simulink library "propertySpecificationOperatorLib"  (Simulink 7.6)
settings: Solver=FixedStepDiscrete  StartTime=0.0  StopTime=10.0  FixedStep=Auto  RelTol=1e-3
libraries: simulink x3, sldvlib x2
settings Model: Creator=itoy  LastModifiedBy=itoy

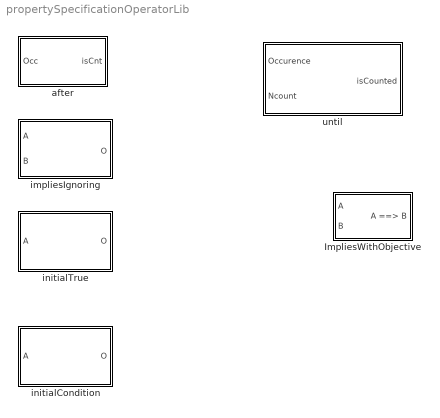
== system propertySpecificationOperatorLib ==
  ImpliesWithObjective : Subsystem
      mask Type: Design Verifier Implies
      mask Description:
      | Tests whether the first input implies the second.  Outputs false
      | when first input is true and second input is false, otherwise
      | outputs true.
      mask Help: helpview(fullfile(docroot,'toolbox','sldv','sldv.map'),'implies')
      mask Display: disp(' ')
  after : Subsystem  mask(After block){TickCount=1}
      mask help:
      | This is an after block.
      | If Occurence are true for successive Ncount time steps, output will be true.
      mask Help: This is a counter block.
      mask Display: fprintf('\nAfter')
  impliesIgnoring : Subsystem  mask{DelayCount=4}
      mask prompts: DelayCount "Delay Count"
      mask Display: fprintf('Implies ignoring\n initial %d steps',DelayCount)
  initialCondition : Subsystem  mask(ignoreInitSteps){DelayCount=4}
      mask prompts: DelayCount "Delay Count"
      mask Display: fprintf('True after \n initial %d steps',DelayCount)
  initialTrue : Subsystem  mask(ignoreInitSteps){DelayCount=5}
      mask prompts: DelayCount "Delay Count"
      mask Display: fprintf('True for \n initial %d steps',DelayCount)
  until : Subsystem  TreatAsAtomicUnit=on
      mask Type: After block
      mask Description:
      | This is an after block.
      | If Occurence are true for successive Ncount time steps, output will be true.
      mask Help: This is a counter block.
      mask Display: fprintf('Until')

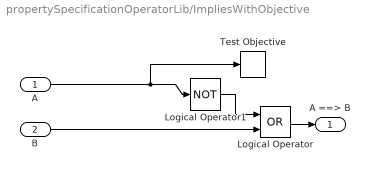
== system propertySpecificationOperatorLib/ImpliesWithObjective ==
  A : Inport
  B : Inport  Port=2
  Logical Operator : Logic  Operator=OR  AllPortsSameDT=off  OutDataTypeStr=boolean
  Logical Operator1 : Logic  Operator=NOT  AllPortsSameDT=off  OutDataTypeStr=boolean
  Test Objective : sldvlib/Test Objective  SystemSampleTime=-1  enabled=on  customAVTBlockType=Test Objective  intervals=true  dispValues=on  outEnabled=off
      settings: AttributesFormatString=%<intervals>
  A ==> B : Outport
  wires:
  Logical Operator1/1 -> Logical Operator/1
  A/1 -> Logical Operator1/1, Test Objective/1
  Logical Operator/1 -> A ==> B/1
  B/1 -> Logical Operator/2

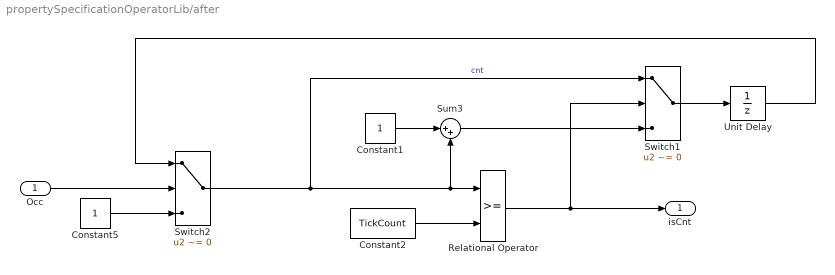
== system propertySpecificationOperatorLib/after ==
  Occ : Inport  OutDataTypeStr=boolean
  Constant1 : Constant  OutDataTypeStr=Inherit: Inherit via back propagation
  Constant2 : Constant  Value=TickCount  OutDataTypeStr=Inherit: Inherit via back propagation
  Constant5 : Constant  OutDataTypeStr=Inherit: Inherit via back propagation
  Relational Operator : RelationalOperator  OutDataTypeStr=boolean
  Sum3 : Sum  Inputs=|++  OutDataTypeStr=Inherit: Inherit via back propagation
  Switch1 : Switch  Criteria=u2 ~= 0  OutDataTypeStr=Inherit: Inherit via back propagation
  Switch2 : Switch  Criteria=u2 ~= 0  OutDataTypeStr=uint8
  Unit Delay : UnitDelay  X0=1  SampleTime=-1
      settings: AttributesFormatString=Init = %<X0>
  isCnt : Outport
  wires:
  Relational Operator/1 -> isCnt/1, Switch1/2
  Constant2/1 -> Relational Operator/2
  Switch2/1 -> Sum3/2, Relational Operator/1, Switch1/1  "cnt"
  Occ/1 -> Switch2/2
  Constant5/1 -> Switch2/3
  Constant1/1 -> Sum3/1
  Unit Delay/1 -> Switch2/1
  Switch1/1 -> Unit Delay/1
  Sum3/1 -> Switch1/3

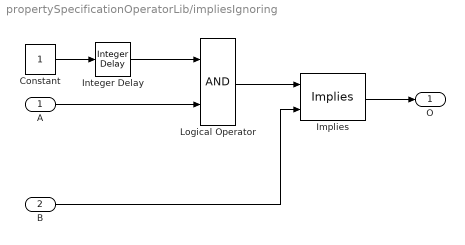
== system propertySpecificationOperatorLib/impliesIgnoring ==
  A : Inport
  B : Inport  Port=2
  Constant : Constant  OutDataTypeStr=boolean
  Implies : sldvlib/Implies  SystemSampleTime=-1
  Integer Delay : simulink/Discrete/Integer Delay  NumDelays=DelayCount  InputProcessing=Inherited  vinit=0  samptime=-1
  Logical Operator : Logic  AllPortsSameDT=off  OutDataTypeStr=boolean
  O : Outport
  wires:
  Implies/1 -> O/1
  Logical Operator/1 -> Implies/1
  Constant/1 -> Integer Delay/1
  Integer Delay/1 -> Logical Operator/1
  A/1 -> Logical Operator/2
  B/1 -> Implies/2

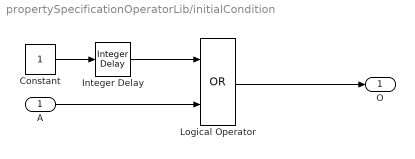
== system propertySpecificationOperatorLib/initialCondition ==
  A : Inport
  Constant : Constant  OutDataTypeStr=boolean
  Integer Delay : simulink/Discrete/Integer Delay  NumDelays=DelayCount  InputProcessing=Inherited  vinit=0  samptime=-1
  Logical Operator : Logic  Operator=OR  AllPortsSameDT=off  OutDataTypeStr=boolean
  O : Outport
  wires:
  Logical Operator/1 -> O/1
  Constant/1 -> Integer Delay/1
  Integer Delay/1 -> Logical Operator/1
  A/1 -> Logical Operator/2

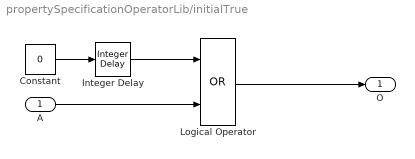
== system propertySpecificationOperatorLib/initialTrue ==
  A : Inport
  Constant : Constant  Value=0  OutDataTypeStr=boolean
  Integer Delay : simulink/Discrete/Integer Delay  NumDelays=DelayCount  InputProcessing=Inherited  vinit=0  samptime=-1
  Logical Operator : Logic  Operator=OR  AllPortsSameDT=off  OutDataTypeStr=boolean
  O : Outport
  wires:
  A/1 -> Logical Operator/2
  Integer Delay/1 -> Logical Operator/1
  Constant/1 -> Integer Delay/1
  Logical Operator/1 -> O/1

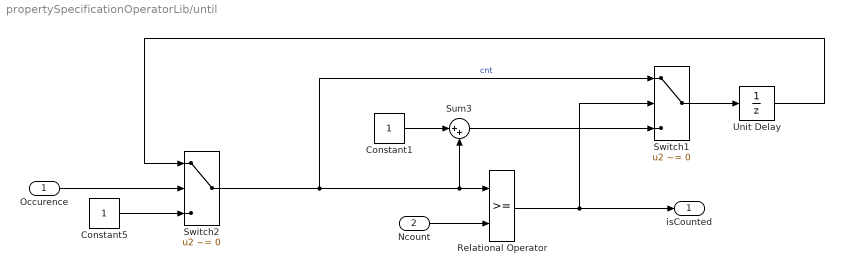
== system propertySpecificationOperatorLib/until ==
  Occurence : Inport  OutDataTypeStr=boolean
  Ncount : Inport  Port=2
  Constant1 : Constant  OutDataTypeStr=Inherit: Inherit via back propagation
  Constant5 : Constant  OutDataTypeStr=Inherit: Inherit via back propagation
  Relational Operator : RelationalOperator  OutDataTypeStr=boolean
  Sum3 : Sum  Inputs=|++  OutDataTypeStr=Inherit: Inherit via back propagation
  Switch1 : Switch  Criteria=u2 ~= 0  OutDataTypeStr=Inherit: Inherit via back propagation
  Switch2 : Switch  Criteria=u2 ~= 0  OutDataTypeStr=uint8
  Unit Delay : UnitDelay  X0=1  SampleTime=-1
      settings: AttributesFormatString=Init = %<X0>
  isCounted : Outport
  wires:
  Sum3/1 -> Switch1/3
  Switch1/1 -> Unit Delay/1
  Unit Delay/1 -> Switch2/1
  Constant1/1 -> Sum3/1
  Constant5/1 -> Switch2/3
  Occurence/1 -> Switch2/2
  Switch2/1 -> Switch1/1, Relational Operator/1, Sum3/2  "cnt"
  Ncount/1 -> Relational Operator/2
  Relational Operator/1 -> Switch1/2, isCounted/1
